simulink model "inner_trans"  (R2018a)
settings: Solver=VariableStepAuto  StartTime=0.0  StopTime=10.0  RelTol=1e-3
settings Model: Creator=BEAR  LastModifiedBy=BEAR

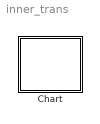
== system inner_trans ==
  Chart : Stateflow chart  TreatAsAtomicUnit=on

== stateflow chart inner_trans/Chart ==
  state super
    en: out=1
    du: out=2
    state sub1
      en: out=7
      ex: out=8
    state sub2
    (default) -> sub1 : {out=3}/{out=4}
    super -> sub1 : {out=5}/{out=6}
    sub1 -> sub2
    sub2 -> sub1
  (default) -> super
  data: out local
